simulink model "FULL_HEART_PICTURE"  (R2023a)
settings: Solver=VariableStepAuto  StartTime=0.0  StopTime=60  RelTol=1e-3  AbsTol=1e-3
libraries: fl_lib x33, sh_lib x18, nesl_utility x6, Cardiovascular_lib x4
settings Model: Creator=luca  LastModifiedBy=Syed Abdul Rahman
settings SolverCC: AutoScaleAbsTol=off  ZeroCrossAlgorithm=Adaptive  AlgebraicLoopSolver=TrustRegion
settings DataIOCC: InspectSignalLogs=on
settings DebuggingCC: IgnoredZcDiagnostic=none  UnconnectedInputMsg=warning  UnconnectedOutputMsg=warning  UnconnectedLineMsg=warning  SymbolicDimsDataTypeCodeGenerationDiagnostic=none
settings ModelReferenceCC: EnableRefExpFcnMdlSchedulingChecks=on
settings SFSimCC: CustomCodeUndefinedFunction=UseInterfaceOnly
settings SimscapeCC: SimscapeLogType=all  SimscapeLogSimulationStatistics=on  SimscapeLogDataHistory=10000

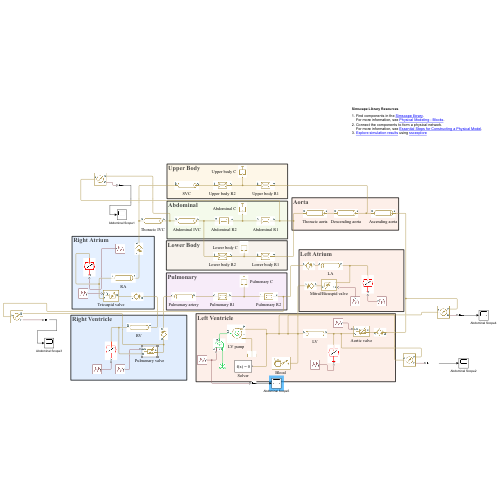
[thumbnail: Simulink's stored preview of the top-level diagram]
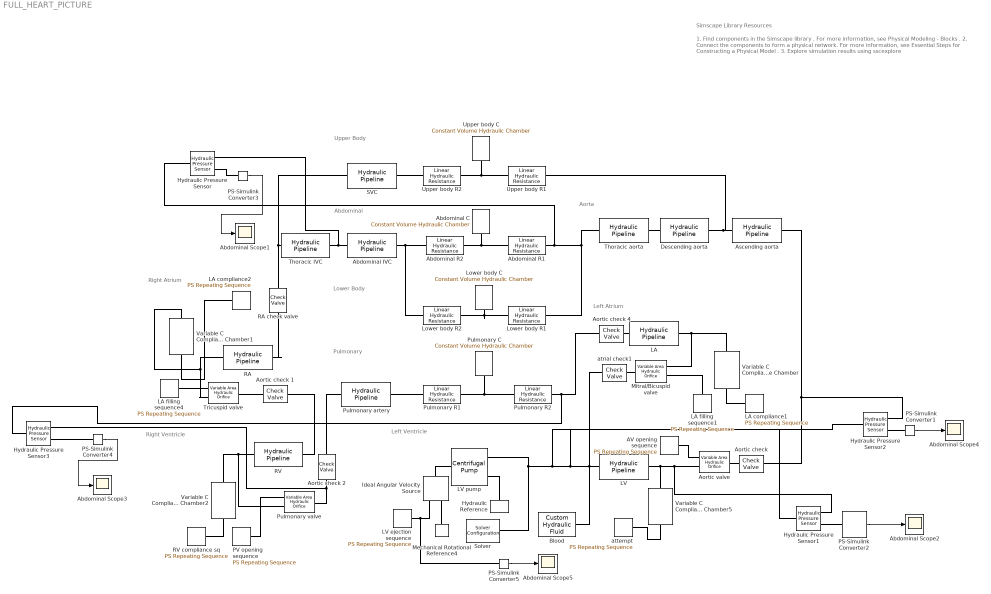
== system FULL_HEART_PICTURE ==
  note: Lower Body
  note: Left Atrium
  note: Right Ventricle
  note: Abdominal
  note: Aorta
  note: 1. Find components in the Simscape library .
      | For more information, see Physical Modeling - Blocks .
      | 2. Connect the components to form a physical network.
      | For more information, see Essential Steps for Constructing a Physical Model .
      | 3. Explore simulation results using sscexplore
  note: Simscape Library Resources
  note: Left Ventricle
  note: Right Atrium
  note: Pulmonary
  note: Upper Body
  AV opening sequence : fl_lib/Physical Signals/Sources/PS Repeating Sequence  y_init=0  offset=0 s  sig_type=2  durations=[0.01 0.01 0.01 0.01 0.01 0.01 0.01 0.01 0.01 0.01 0.01 0.01 0.01 0.01 0.01 0.01 0.01 0.01 0.01 0.01 0.01 0.01 0.01 0.01 0.01 0.01 0.01 0.01 0.01 0.01 0.01 0.01 0.01 0.01 0.01 0.01 0.01 0.01 0.01 0.01 0.01 0.01 0.01 0.01 0.01 0.01 0.01 0.01 0.01 0.01 0.01 0.01 0.01 0.01 0.01 0.01 0.01 0.01 0.01 0.01 0.01 0.01 0.01 0.01 0.01 0.01 0.01 0.01 0.01 0.01 0.01 0.01 0.01 0.01 0.01 0.01 0.01 0.01 0.01 0.01 0.01 0.01 0.01 0.01 0.01 0.01 0.01 0.01 0.01 0.01 0.01 0.01 0.01 0.01 0.01 0.01 0.01 0.01 0.01 0.01] s  y_start="[0.000300000000000000\t0.000300000000000000\t0.000300000000000000\t0.000300000000000000\t0.000300000000000000\t0.000300000000000000\t0.000300000000000000\t0.000300000000000000\t0.000300000000000000\t0.000300000000000000\t0.000300000000000000\t0.000300000000000000\t0.000300000000000000\t0.000300000000000000\t0.000300000000000000\t0.000300000000000000\t0.000300000000000000\t0.000300000000000000\t0.000300000000000000\t0.000300000000000000\t0.000300000000000000\t0.000300000000000000\t0.000300000000000000\t0.000300000000000000\t0.000300000000000000\t0.000300000000000000\t0.000300000000000000\t0.000300000000000000\t0.000300000000000000\t0.000300000000000000\t0.000300000000000000\t0.000300000000000000\t0.000300000000000000\t0.000300000000000000\t0.000300000000000000\t0.000300000000000000\t0.000300000000000000\t0.000300000000000000\t0.000300000000000000\t0.000300000000000000\t0.000300000000000000\t0.000300000000000000\t0.000300000000000000\t0\t0\t0\t0\t0\t0\t0\t0\t0\t0\t0\t0\t0\t0\t0\t0\t0\t0\t0\t0\t0\t0\t0\t0\t0\t0\t0\t0\t0\t0\t0\t0\t0\t0\t0\t0\t0\t0\t0\t0\t0\t0\t0\t0\t0\t0\t0\t0\t0\t0\t0\t0\t0\t0\t0\t0\t0]/3*4"  y_end=1
      settings: InternalSimscapePortConfiguration="{\"Bottom\":[],\"Left\":[],\"Right\":[{\"id\":\"Y\",\"label\":\"Y\",\"type\":\"output\"}],\"Top\":[]}"
  Abdominal C : fl_lib/Hydraulic/Hydraulic Elements/Constant Volume Hydraulic Chamber  ch_sp=2  wall_type=2  ch_volume=1e-4 m^3  d_in=1 cm  length=2570.700637 cm  pr_r_coef=3.6E-08 m/Pa  time_const=0.01 s  k_sh=1.4  pressure_specify=off  pressure_priority=High  pressure=0 Pa  pressure_nominal_specify=off  pressure_nominal_unit=Pa  pressure_nominal_value=1  diameter_incr_specify=off  diameter_incr_priority=High  diameter_incr=0 m  diameter_incr_nominal_specify=off  diameter_incr_nominal_unit=m  diameter_incr_nominal_value=1  flow_rate_specify=off  flow_rate_priority=None  flow_rate=0.001 m^3/s  flow_rate_nominal_specify=off  flow_rate_nominal_unit=m^3/s  flow_rate_nominal_value=1
      settings: InternalSimscapePortConfiguration="{\"Bottom\":[],\"Left\":[{\"id\":\"A\",\"label\":\"\",\"type\":\"foundation.hydraulic.hydraulic\"}],\"Right\":[],\"Top\":[]}"
  Abdominal IVC : sh_lib/Pipelines/Hydraulic Pipeline  cs_type=1  d_in=1.37 cm  area=1e-4 m^2  D_h=1.12e-2 m  s_factor=64  length=17 cm  length_ad=0 m  roughness=15e-6 m  Re_lam=2000  Re_turb=4000  wall_type=2  pr_r_coef=4.39e-6 m/Pa  time_const=0.01 s  k_sh=1.4  initial_pressure=0 Pa
      settings: InternalSimscapePortConfiguration="{\"Bottom\":[],\"Left\":[{\"id\":\"A\",\"label\":\"A\",\"type\":\"foundation.hydraulic.hydraulic\"}],\"Right\":[{\"id\":\"B\",\"label\":\"B\",\"type\":\"foundation.hydraulic.hydraulic\"}],\"Top\":[]}"
  Abdominal R1 : fl_lib/Hydraulic/Hydraulic Elements/Linear Hydraulic Resistance  resistance=2.3e8 Pa/(m^3/s)  q_specify=off  q_priority=None  q=0.001 m^3/s  q_nominal_specify=off  q_nominal_unit=m^3/s  q_nominal_value=1  p_specify=off  p_priority=None  p=0 Pa  p_nominal_specify=off  p_nominal_unit=Pa  p_nominal_value=1
      settings: InternalSimscapePortConfiguration="{\"Bottom\":[],\"Left\":[{\"id\":\"A\",\"label\":\"A\",\"type\":\"foundation.hydraulic.hydraulic\"}],\"Right\":[{\"id\":\"B\",\"label\":\"B\",\"type\":\"foundation.hydraulic.hydraulic\"}],\"Top\":[]}"
  Abdominal R2 : fl_lib/Hydraulic/Hydraulic Elements/Linear Hydraulic Resistance  resistance=0.15e8 Pa/(m^3/s)  q_specify=off  q_priority=None  q=0.001 m^3/s  q_nominal_specify=off  q_nominal_unit=m^3/s  q_nominal_value=1  p_specify=off  p_priority=None  p=0 Pa  p_nominal_specify=off  p_nominal_unit=Pa  p_nominal_value=1
      settings: InternalSimscapePortConfiguration="{\"Bottom\":[],\"Left\":[{\"id\":\"A\",\"label\":\"A\",\"type\":\"foundation.hydraulic.hydraulic\"}],\"Right\":[{\"id\":\"B\",\"label\":\"B\",\"type\":\"foundation.hydraulic.hydraulic\"}],\"Top\":[]}"
  Abdominal Scope{1..5} (5 alike) : Scope
  "Aortic check " : sh_lib/Valves/Directional Valves/Check Valve  area_max=1e-1 m^2  pres_crack=0.01 Pa  pres_max=0.1 Pa  C_d=1  A_leak=1e-12 m^2  lam_spec=1  B_lam=0.999  Re_cr=12  dynamic=0  tau=0.1 s  area_init=1e-12 m^2
      settings: InternalSimscapePortConfiguration="{\"Bottom\":[],\"Left\":[{\"id\":\"A\",\"label\":\"A\",\"type\":\"foundation.hydraulic.hydraulic\"}],\"Right\":[{\"id\":\"B\",\"label\":\"B\",\"type\":\"foundation.hydraulic.hydraulic\"}],\"Top\":[]}"
  Aortic check 1 : sh_lib/Valves/Directional Valves/Check Valve  area_max=1e-1 m^2  pres_crack=0.01 Pa  pres_max=0.1 Pa  C_d=1  A_leak=1e-12 m^2  lam_spec=1  B_lam=0.999  Re_cr=12  dynamic=0  tau=0.1 s  area_init=1e-12 m^2
      settings: InternalSimscapePortConfiguration="{\"Bottom\":[],\"Left\":[{\"id\":\"A\",\"label\":\"A\",\"type\":\"foundation.hydraulic.hydraulic\"}],\"Right\":[{\"id\":\"B\",\"label\":\"B\",\"type\":\"foundation.hydraulic.hydraulic\"}],\"Top\":[]}"
  Aortic check 2 : sh_lib/Valves/Directional Valves/Check Valve  area_max=1e-1 m^2  pres_crack=0.01 Pa  pres_max=0.1 Pa  C_d=1  A_leak=1e-12 m^2  lam_spec=1  B_lam=0.999  Re_cr=12  dynamic=0  tau=0.1 s  area_init=1e-12 m^2
      settings: InternalSimscapePortConfiguration="{\"Bottom\":[],\"Left\":[{\"id\":\"A\",\"label\":\"A\",\"type\":\"foundation.hydraulic.hydraulic\"}],\"Right\":[{\"id\":\"B\",\"label\":\"B\",\"type\":\"foundation.hydraulic.hydraulic\"}],\"Top\":[]}"
  Aortic check 4 : sh_lib/Valves/Directional Valves/Check Valve  area_max=1e-3 m^2  pres_crack=0.01 Pa  pres_max=0.1 Pa  C_d=1  A_leak=1e-12 m^2  lam_spec=1  B_lam=0.999  Re_cr=12  dynamic=0  tau=0.1 s  area_init=1e-12 m^2
      settings: InternalSimscapePortConfiguration="{\"Bottom\":[],\"Left\":[{\"id\":\"A\",\"label\":\"A\",\"type\":\"foundation.hydraulic.hydraulic\"}],\"Right\":[{\"id\":\"B\",\"label\":\"B\",\"type\":\"foundation.hydraulic.hydraulic\"}],\"Top\":[]}"
  Aortic valve : fl_lib/Hydraulic/Hydraulic Elements/Variable Area Hydraulic Orifice  C_d=1  min_area=1e-15 m^2  lam_spec=1  B_lam=0.999  Re_cr=12  q_specify=off  q_priority=None  q=0.001 m^3/s  q_nominal_specify=off  q_nominal_unit=m^3/s  q_nominal_value=1  p_specify=off  p_priority=None  p=0 Pa  p_nominal_specify=off  p_nominal_unit=Pa  p_nominal_value=1
      settings: InternalSimscapePortConfiguration="{\"Bottom\":[],\"Left\":[{\"id\":\"AR\",\"label\":\"AR\",\"type\":\"input\"},{\"id\":\"A\",\"label\":\"A\",\"type\":\"foundation.hydraulic.hydraulic\"}],\"Right\":[{\"id\":\"B\",\"label\":\"B\",\"type\":\"foundation.hydraulic.hydraulic\"}],\"Top\":[]}"
  Ascending aorta : sh_lib/Pipelines/Hydraulic Pipeline  cs_type=1  d_in=2.65 cm  area=1e-4 m^2  D_h=1.12e-2 m  s_factor=64  length=8.8 cm  length_ad=0 m  roughness=15e-6 m  Re_lam=2000  Re_turb=4000  wall_type=2  pr_r_coef=4.5e-7 m/Pa  time_const=0.01 s  k_sh=1.4  initial_pressure=0 Pa
      settings: InternalSimscapePortConfiguration="{\"Bottom\":[],\"Left\":[{\"id\":\"A\",\"label\":\"A\",\"type\":\"foundation.hydraulic.hydraulic\"}],\"Right\":[{\"id\":\"B\",\"label\":\"B\",\"type\":\"foundation.hydraulic.hydraulic\"}],\"Top\":[]}"
  "Blood " : fl_lib/Hydraulic/Hydraulic Utilities/Custom Hydraulic Fluid  density=1060 kg/m^3  viscosity_kin=3.55e-6 m^2/s  bulk=2.2e9 Pa  alpha=0.005  range_error=2
      settings: InternalSimscapePortConfiguration="{\"Bottom\":[],\"Left\":[],\"Right\":[{\"id\":\"G\",\"label\":\"\",\"type\":\"foundation.hydraulic.hydraulic\"}],\"Top\":[]}"
  Descending aorta : sh_lib/Pipelines/Hydraulic Pipeline  cs_type=1  d_in=2.15 cm  area=1e-4 m^2  D_h=1.12e-2 m  s_factor=64  length=6.94 cm  length_ad=0 m  roughness=15e-6 m  Re_lam=2000  Re_turb=4000  wall_type=2  pr_r_coef=1.4e-6 m/Pa  time_const=0.01 s  k_sh=1.4  initial_pressure=0 Pa
      settings: InternalSimscapePortConfiguration="{\"Bottom\":[],\"Left\":[{\"id\":\"A\",\"label\":\"A\",\"type\":\"foundation.hydraulic.hydraulic\"}],\"Right\":[{\"id\":\"B\",\"label\":\"B\",\"type\":\"foundation.hydraulic.hydraulic\"}],\"Top\":[]}"
  Hydraulic Pressure Sensor{,1..3} (4 alike) : fl_lib/Hydraulic/Hydraulic Sensors/Hydraulic Pressure Sensor
  Hydraulic Reference : fl_lib/Hydraulic/Hydraulic Elements/Hydraulic Reference
  Ideal Angular Velocity Source : fl_lib/Mechanical/Mechanical Sources/Ideal Angular Velocity Source
  LA : sh_lib/Pipelines/Hydraulic Pipeline  cs_type=1  d_in=4.8 cm  area=1e-4 m^2  D_h=1.12e-2 m  s_factor=64  length=5 cm  length_ad=0 m  roughness=15e-6 m  Re_lam=2000  Re_turb=4000  wall_type=1  pr_r_coef=5.9e-6 m/Pa  time_const=0.01 s  k_sh=1.4  initial_pressure=0 Pa
      settings: InternalSimscapePortConfiguration="{\"Bottom\":[],\"Left\":[{\"id\":\"A\",\"label\":\"A\",\"type\":\"foundation.hydraulic.hydraulic\"}],\"Right\":[{\"id\":\"B\",\"label\":\"B\",\"type\":\"foundation.hydraulic.hydraulic\"}],\"Top\":[]}"
  LA compliance1 : fl_lib/Physical Signals/Sources/PS Repeating Sequence  y_init=0  offset=0 s  sig_type=2  durations=[0.01 0.01 0.01 0.01 0.01 0.01 0.01 0.01 0.01 0.01 0.01 0.01 0.01 0.01 0.01 0.01 0.01 0.01 0.01 0.01 0.01 0.01 0.01 0.01 0.01 0.01 0.01 0.01 0.01 0.01 0.01 0.01 0.01 0.01 0.01 0.01 0.01 0.01 0.01 0.01 0.01 0.01 0.01 0.01 0.01 0.01 0.01 0.01 0.01 0.01 0.01 0.01 0.01 0.01 0.01 0.01 0.01 0.01 0.01 0.01 0.01 0.01 0.01 0.01 0.01 0.01 0.01 0.01 0.01 0.01 0.01 0.01 0.01 0.01 0.01 0.01 0.01 0.01 0.01 0.01 0.01 0.01 0.01 0.01 0.01 0.01 0.01 0.01 0.01 0.01 0.01 0.01 0.01 0.01 0.01 0.01 0.01 0.01 0.01 0.01] s  y_start="[1.36500000000000e-05\t1.36862500000000e-05\t1.37225000000000e-05\t1.37587500000000e-05\t1.37950000000000e-05\t1.38312500000000e-05\t1.38675000000000e-05\t1.39037500000000e-05\t1.39400000000000e-05\t1.39762500000000e-05\t1.40125000000000e-05\t1.40487500000000e-05\t1.40850000000000e-05\t1.41212500000000e-05\t1.41575000000000e-05\t1.41937500000000e-05\t1.42300000000000e-05\t1.42662500000000e-05\t1.43025000000000e-05\t1.43387500000000e-05\t1.43750000000000e-05\t1.44112500000000e-05\t1.44475000000000e-05\t1.44837500000000e-05\t1.45200000000000e-05\t1.45562500000000e-05\t1.45925000000000e-05\t1.46287500000000e-05\t1.46650000000000e-05\t1.47012500000000e-05\t1.47375000000000e-05\t1.47737500000000e-05\t1.48100000000000e-05\t1.48462500000000e-05\t1.48825000000000e-05\t1.49187500000000e-05\t1.49550000000000e-05\t1.49912500000000e-05\t1.50275000000000e-05\t1.50637500000000e-05\t1.51000000000000e-05\t1.51362500000000e-05\t1.51725000000000e-05\t1.52087500000000e-05\t1.52450000000000e-05\t1.52812500000000e-05\t1.53175000000000e-05\t1.53537500000000e-05\t1.53900000000000e-05\t1.54262500000000e-05\t1.54625000000000e-05\t1.54987500000000e-05\t1.55350000000000e-05\t1.55712500000000e-05\t1.56075000000000e-05\t1.56437500000000e-05\t1.56800000000000e-05\t1.57162500000000e-05\t1.57525000000000e-05\t1.57887500000000e-05\t1.58250000000000e-05\t1.58612500000000e-05\t1.58975000000000e-05\t1.59337500000000e-05\t1.59700000000000e-05\t1.60062500000000e-05\t1.60425000000000e-05\t1.60787500000000e-05\t1.61150000000000e-05\t1.61512500000000e-05\t1.61875000000000e-05\t1.62237500000000e-05\t1.62600000000000e-05\t1.62962500000000e-05\t1.63325000000000e-05\t1.63687500000000e-05\t1.64050000000000e-05\t1.64412500000000e-05\t1.64775000000000e-05\t1.65137500000000e-05\t1.36500000000000e-05\t1.29125270139567e-05\t1.21876723951708e-05\t1.14878386071372e-05\t1.08250000000000e-05\t1.02104979261007e-05\t9.65484668629601e-06\t9.16755362735452e-06\t8.75695646861792e-06\t8.43008064131123e-06\t8.19251908146676e-06\t8.04833653323797e-06\t8.00000000000000e-06\t8.14165729617270e-06\t8.55952589635133e-06\t9.23265212405563e-06\t1.01272826194982e-05\t1.11985568739858e-05\t1.23927567231468e-05\t1.36500000000000e-05]"  y_end=1
      settings: InternalSimscapePortConfiguration="{\"Bottom\":[],\"Left\":[],\"Right\":[{\"id\":\"Y\",\"label\":\"Y\",\"type\":\"output\"}],\"Top\":[]}"
  LA compliance2 : fl_lib/Physical Signals/Sources/PS Repeating Sequence  y_init=0  offset=0 s  sig_type=2  durations=[0.01 0.01 0.01 0.01 0.01 0.01 0.01 0.01 0.01 0.01 0.01 0.01 0.01 0.01 0.01 0.01 0.01 0.01 0.01 0.01 0.01 0.01 0.01 0.01 0.01 0.01 0.01 0.01 0.01 0.01 0.01 0.01 0.01 0.01 0.01 0.01 0.01 0.01 0.01 0.01 0.01 0.01 0.01 0.01 0.01 0.01 0.01 0.01 0.01 0.01 0.01 0.01 0.01 0.01 0.01 0.01 0.01 0.01 0.01 0.01 0.01 0.01 0.01 0.01 0.01 0.01 0.01 0.01 0.01 0.01 0.01 0.01 0.01 0.01 0.01 0.01 0.01 0.01 0.01 0.01 0.01 0.01 0.01 0.01 0.01 0.01 0.01 0.01 0.01 0.01 0.01 0.01 0.01 0.01 0.01 0.01 0.01 0.01 0.01 0.01] s  y_start="[2.18400000000000e-05\t2.18580000000000e-05\t2.18760000000000e-05\t2.18940000000000e-05\t2.19120000000000e-05\t2.19300000000000e-05\t2.19480000000000e-05\t2.19660000000000e-05\t2.19840000000000e-05\t2.20020000000000e-05\t2.20200000000000e-05\t2.20380000000000e-05\t2.20560000000000e-05\t2.20740000000000e-05\t2.20920000000000e-05\t2.21100000000000e-05\t2.21280000000000e-05\t2.21460000000000e-05\t2.21640000000000e-05\t2.21820000000000e-05\t2.22000000000000e-05\t2.22180000000000e-05\t2.22360000000000e-05\t2.22540000000000e-05\t2.22720000000000e-05\t2.22900000000000e-05\t2.23080000000000e-05\t2.23260000000000e-05\t2.23440000000000e-05\t2.23620000000000e-05\t2.23800000000000e-05\t2.23980000000000e-05\t2.24160000000000e-05\t2.24340000000000e-05\t2.24520000000000e-05\t2.24700000000000e-05\t2.24880000000000e-05\t2.25060000000000e-05\t2.25240000000000e-05\t2.25420000000000e-05\t2.25600000000000e-05\t2.25780000000000e-05\t2.25960000000000e-05\t2.26140000000000e-05\t2.26320000000000e-05\t2.26500000000000e-05\t2.26680000000000e-05\t2.26860000000000e-05\t2.27040000000000e-05\t2.27220000000000e-05\t2.27400000000000e-05\t2.27580000000000e-05\t2.27760000000000e-05\t2.27940000000000e-05\t2.28120000000000e-05\t2.28300000000000e-05\t2.28480000000000e-05\t2.28660000000000e-05\t2.28840000000000e-05\t2.29020000000000e-05\t2.29200000000000e-05\t2.29380000000000e-05\t2.29560000000000e-05\t2.29740000000000e-05\t2.29920000000000e-05\t2.30100000000000e-05\t2.30280000000000e-05\t2.30460000000000e-05\t2.30640000000000e-05\t2.30820000000000e-05\t2.31000000000000e-05\t2.31180000000000e-05\t2.31360000000000e-05\t2.31540000000000e-05\t2.31720000000000e-05\t2.31900000000000e-05\t2.32080000000000e-05\t2.32260000000000e-05\t2.32440000000000e-05\t2.32620000000000e-05\t2.18400000000000e-05\t2.14693056140951e-05\t2.11049539119088e-05\t2.07531790520831e-05\t2.04200000000000e-05\t2.01111175416152e-05\t1.98318167414302e-05\t1.95868765135729e-05\t1.93804878532522e-05\t1.92161821276679e-05\t1.90967706533390e-05\t1.90242965936984e-05\t1.90000000000000e-05\t1.90712047294036e-05\t1.92812484151571e-05\t1.96195985897908e-05\t2.00692889627212e-05\t2.06077701809061e-05\t2.12080405475641e-05\t2.18400000000000e-05]"  y_end=1
      settings: InternalSimscapePortConfiguration="{\"Bottom\":[],\"Left\":[],\"Right\":[{\"id\":\"Y\",\"label\":\"Y\",\"type\":\"output\"}],\"Top\":[]}"
  LA filling sequence1 : fl_lib/Physical Signals/Sources/PS Repeating Sequence  y_init=0  offset=0 s  sig_type=2  durations=[0.01 0.01 0.01 0.01 0.01 0.01 0.01 0.01 0.01 0.01 0.01 0.01 0.01 0.01 0.01 0.01 0.01 0.01 0.01 0.01 0.01 0.01 0.01 0.01 0.01 0.01 0.01 0.01 0.01 0.01 0.01 0.01 0.01 0.01 0.01 0.01 0.01 0.01 0.01 0.01 0.01 0.01 0.01 0.01 0.01 0.01 0.01 0.01 0.01 0.01 0.01 0.01 0.01 0.01 0.01 0.01 0.01 0.01 0.01 0.01 0.01 0.01 0.01 0.01 0.01 0.01 0.01 0.01 0.01 0.01 0.01 0.01 0.01 0.01 0.01 0.01 0.01 0.01 0.01 0.01 0.01 0.01 0.01 0.01 0.01 0.01 0.01 0.01 0.01 0.01 0.01 0.01 0.01 0.01 0.01 0.01 0.01 0.01 0.01 0.01] s  y_start="[0\t0\t0\t0\t0\t0\t0\t0\t0\t0\t0\t0\t0\t0\t0\t0\t0\t0\t0\t0\t0\t0\t0\t0\t0\t0\t0\t0\t0\t0\t0\t0\t0\t0\t0\t0\t0\t0\t0\t0\t0\t0\t0\t0\t0\t0.000420000000000000\t0.000420000000000000\t0.000420000000000000\t0.000420000000000000\t0.000420000000000000\t0.000420000000000000\t0.000420000000000000\t0.000420000000000000\t0.000420000000000000\t0.000420000000000000\t0.000420000000000000\t0.000420000000000000\t0.000420000000000000\t0.000420000000000000\t0.000420000000000000\t0.000420000000000000\t0.000420000000000000\t0.000420000000000000\t0.000420000000000000\t0.000420000000000000\t0.000420000000000000\t0.000420000000000000\t0.000420000000000000\t0.000420000000000000\t0.000420000000000000\t0.000420000000000000\t0.000420000000000000\t0.000420000000000000\t0.000420000000000000\t0.000420000000000000\t0.000420000000000000\t0.000420000000000000\t0.000420000000000000\t0.000420000000000000\t0.000420000000000000\t0.000420000000000000\t0.000420000000000000\t0.000420000000000000\t0.000420000000000000\t0.000420000000000000\t0.000420000000000000\t0.000420000000000000\t0.000420000000000000\t0.000420000000000000\t0.000420000000000000\t0.000420000000000000\t0.000420000000000000\t0.000420000000000000\t0.000420000000000000\t0.000420000000000000\t0.000420000000000000\t0.000420000000000000\t0.000420000000000000\t0.000420000000000000\t0.000420000000000000]"  y_end=1
      settings: InternalSimscapePortConfiguration="{\"Bottom\":[],\"Left\":[],\"Right\":[{\"id\":\"Y\",\"label\":\"Y\",\"type\":\"output\"}],\"Top\":[]}"
  LA filling sequence4 : fl_lib/Physical Signals/Sources/PS Repeating Sequence  y_init=0  offset=0 s  sig_type=2  durations=[0.01 0.01 0.01 0.01 0.01 0.01 0.01 0.01 0.01 0.01 0.01 0.01 0.01 0.01 0.01 0.01 0.01 0.01 0.01 0.01 0.01 0.01 0.01 0.01 0.01 0.01 0.01 0.01 0.01 0.01 0.01 0.01 0.01 0.01 0.01 0.01 0.01 0.01 0.01 0.01 0.01 0.01 0.01 0.01 0.01 0.01 0.01 0.01 0.01 0.01 0.01 0.01 0.01 0.01 0.01 0.01 0.01 0.01 0.01 0.01 0.01 0.01 0.01 0.01 0.01 0.01 0.01 0.01 0.01 0.01 0.01 0.01 0.01 0.01 0.01 0.01 0.01 0.01 0.01 0.01 0.01 0.01 0.01 0.01 0.01 0.01 0.01 0.01 0.01 0.01 0.01 0.01 0.01 0.01 0.01 0.01 0.01 0.01 0.01 0.01] s  y_start="[0\t0\t0\t0\t0\t0\t0\t0\t0\t0\t0\t0\t0\t0\t0\t0\t0\t0\t0\t0\t0\t0\t0\t0\t0\t0\t0\t0\t0\t0\t0\t0\t0\t0\t0\t0\t0\t0\t0\t0\t0\t0\t0\t0\t0\t0.000500000000000000\t0.000500000000000000\t0.000500000000000000\t0.000500000000000000\t0.000500000000000000\t0.000500000000000000\t0.000500000000000000\t0.000500000000000000\t0.000500000000000000\t0.000500000000000000\t0.000500000000000000\t0.000500000000000000\t0.000500000000000000\t0.000500000000000000\t0.000500000000000000\t0.000500000000000000\t0.000500000000000000\t0.000500000000000000\t0.000500000000000000\t0.000500000000000000\t0.000500000000000000\t0.000500000000000000\t0.000500000000000000\t0.000500000000000000\t0.000500000000000000\t0.000500000000000000\t0.000500000000000000\t0.000500000000000000\t0.000500000000000000\t0.000500000000000000\t0.000500000000000000\t0.000500000000000000\t0.000500000000000000\t0.000500000000000000\t0.000500000000000000\t0.000500000000000000\t0.000500000000000000\t0.000500000000000000\t0.000500000000000000\t0.000500000000000000\t0.000500000000000000\t0.000500000000000000\t0.000500000000000000\t0.000500000000000000\t0.000500000000000000\t0.000500000000000000\t0.000500000000000000\t0.000500000000000000\t0.000500000000000000\t0.000500000000000000\t0.000500000000000000\t0.000500000000000000\t0.000500000000000000\t0.000500000000000000\t0.000500000000000000]"  y_end=1
      settings: InternalSimscapePortConfiguration="{\"Bottom\":[],\"Left\":[],\"Right\":[{\"id\":\"Y\",\"label\":\"Y\",\"type\":\"output\"}],\"Top\":[]}"
  LV : sh_lib/Pipelines/Hydraulic Pipeline  cs_type=1  d_in=4.4 cm  area=1e-4 m^2  D_h=1.12e-2 m  s_factor=64  length=7 cm  length_ad=0 m  roughness=15e-6 m  Re_lam=2000  Re_turb=4000  wall_type=1  pr_r_coef=3.8e-7 m/Pa  time_const=0.01 s  k_sh=1.4  initial_pressure=0 Pa
      settings: InternalSimscapePortConfiguration="{\"Bottom\":[],\"Left\":[{\"id\":\"A\",\"label\":\"A\",\"type\":\"foundation.hydraulic.hydraulic\"}],\"Right\":[{\"id\":\"B\",\"label\":\"B\",\"type\":\"foundation.hydraulic.hydraulic\"}],\"Top\":[]}"
  LV ejection sequence : fl_lib/Physical Signals/Sources/PS Repeating Sequence  y_init=0  offset=0 s  sig_type=2  durations=[0.01 0.01 0.01 0.01 0.01 0.01 0.01 0.01 0.01 0.01 0.01 0.01 0.01 0.01 0.01 0.01 0.01 0.01 0.01 0.01 0.01 0.01 0.01 0.01 0.01 0.01 0.01 0.01 0.01 0.01 0.01 0.01 0.01 0.01 0.01 0.01 0.01 0.01 0.01 0.01 0.01 0.01 0.01 0.01 0.01 0.01 0.01 0.01 0.01 0.01 0.01 0.01 0.01 0.01 0.01 0.01 0.01 0.01 0.01 0.01 0.01 0.01 0.01 0.01 0.01 0.01 0.01 0.01 0.01 0.01 0.01 0.01 0.01 0.01 0.01 0.01 0.01 0.01 0.01 0.01 0.01 0.01 0.01 0.01 0.01 0.01 0.01 0.01 0.01 0.01 0.01 0.01 0.01 0.01 0.01 0.01 0.01 0.01 0.01 0.01] s  y_start=[26.89 53.68 80.24 106.49 132.30 157.58 182.23 206.15 229.23 251.39 272.54 292.59 311.47 329.09 345.38 360.28 373.74 385.68 396.08 404.88 412.05 417.56 421.39 423.52 423.95 422.670 419.68 415.01 408.67 400.68 391.08 379.90 367.19 353.01 337.4 320.44 302.18 282.71 262.1 240.43 217.80 194.29 169.99 145.02 119.45 93.41 66.99 40.3 13.45 0 0 0 0 0 0 0 0 0 0 0 0 0 0 0 0 0 0 0 0 0 0 0 0 0 0 0 0 0 0 0 0 0 0 0 0 0 0 0 0 0 0 0 0 0 0 0 0 0 0 0]*1.15e-1  y_end=1
      settings: InternalSimscapePortConfiguration="{\"Bottom\":[],\"Left\":[],\"Right\":[{\"id\":\"Y\",\"label\":\"Y\",\"type\":\"output\"}],\"Top\":[]}"
  LV pump : sh_lib/Pumps and Motors/Centrifugal Pump  mdl_type=1  c_1=326.8 Pa/(kg/m^3)  c_2=3.104e4 Pa*s/kg  c_3=1.097e7 Pa*s^2/(kg*m^3)  c_4=2.136e5 Pa*s^2/(kg*m^3)  c_f=0.8  design_del=130 lpm  ref_velocity=1770 rpm  ref_density=1060 kg/m^3  leak_resistance=7e6 Pa/(m^3/s)  T_const=0.1 N*m  trq_press_coeff=0.1e-5 N*m/Pa  pump_del_1D=[0, 28, 90, 130, 154, 182] lpm  press_diff_1D=[2.6, 2.4, 2, 1.6, 1.2, .8] bar  pump_del_power_1D=[0, 20, 40, 60, 80, 100, 120, 140, 160] lpm  power_1D=[220, 280, 310, 360, 390, 420, 480, 500, 550] W  pump_vel_2D=[3200, 3300, 3400, 3500] rpm  pump_del_2D=[0, 50, 100, 150, 200, 250, 300, 350] lpm  press_diff_2D=[8.3, 8.8, 9.3, 9.9; 7.8, 8.3, 8.8, 9.4; 7.2, 7.6, 8.2, 8.7; 6.5, 7, 7.5, 8; 5.6, 6.1, 6.6, 7.1; 4.7, 5.2, 5.7, 6.2; 3.4, 4, 4.4, 4.9; 2.3, 2.7, 3.4, 3.6] bar  pump_del_power_2D=[0, 50, 100, 150, 200, 250, 300, 350] lpm  power_2D=[1223, 1341, 1467, 1600; 1414, 1551, 1696, 1850; 1636, 1794, 1962, 2140; 1941, 2129, 2326, 2540; 2224, 2439, 2660, 2910; 2453, 2691, 2947, 3210; 2757, 3024, 3307, 3608; 2945, 3230, 3533, 3854] W  omega_threshold=1e-9 rad/s  interp_method=1  extrap_method=1
      settings: InternalSimscapePortConfiguration="{\"Bottom\":[],\"Left\":[{\"id\":\"S\",\"label\":\"S\",\"type\":\"foundation.mechanical.rotational.rotational\"}],\"Right\":[{\"id\":\"P\",\"label\":\"P\",\"type\":\"foundation.hydraulic.hydraulic\"},{\"id\":\"T\",\"label\":\"T\",\"type\":\"foundation.hydraulic.hydraulic\"}],\"Top\":[]}"
  Lower body C : fl_lib/Hydraulic/Hydraulic Elements/Constant Volume Hydraulic Chamber  ch_sp=2  wall_type=2  ch_volume=1e-4 m^3  d_in=1 cm  length=648.4076433 cm  pr_r_coef=4.1E-08 m/Pa  time_const=0.01 s  k_sh=1.4  pressure_specify=off  pressure_priority=High  pressure=0 Pa  pressure_nominal_specify=off  pressure_nominal_unit=Pa  pressure_nominal_value=1  diameter_incr_specify=off  diameter_incr_priority=High  diameter_incr=0 m  diameter_incr_nominal_specify=off  diameter_incr_nominal_unit=m  diameter_incr_nominal_value=1  flow_rate_specify=off  flow_rate_priority=None  flow_rate=0.001 m^3/s  flow_rate_nominal_specify=off  flow_rate_nominal_unit=m^3/s  flow_rate_nominal_value=1
      settings: InternalSimscapePortConfiguration="{\"Bottom\":[],\"Left\":[{\"id\":\"A\",\"label\":\"\",\"type\":\"foundation.hydraulic.hydraulic\"}],\"Right\":[],\"Top\":[]}"
  Lower body R1 : fl_lib/Hydraulic/Hydraulic Elements/Linear Hydraulic Resistance  resistance=4.79e8 Pa/(m^3/s)  q_specify=off  q_priority=None  q=0.001 m^3/s  q_nominal_specify=off  q_nominal_unit=m^3/s  q_nominal_value=1  p_specify=off  p_priority=None  p=0 Pa  p_nominal_specify=off  p_nominal_unit=Pa  p_nominal_value=1
      settings: InternalSimscapePortConfiguration="{\"Bottom\":[],\"Left\":[{\"id\":\"A\",\"label\":\"A\",\"type\":\"foundation.hydraulic.hydraulic\"}],\"Right\":[{\"id\":\"B\",\"label\":\"B\",\"type\":\"foundation.hydraulic.hydraulic\"}],\"Top\":[]}"
  Lower body R2 : fl_lib/Hydraulic/Hydraulic Elements/Linear Hydraulic Resistance  resistance=0.4e8 Pa/(m^3/s)  q_specify=off  q_priority=None  q=0.001 m^3/s  q_nominal_specify=off  q_nominal_unit=m^3/s  q_nominal_value=1  p_specify=off  p_priority=None  p=0 Pa  p_nominal_specify=off  p_nominal_unit=Pa  p_nominal_value=1
      settings: InternalSimscapePortConfiguration="{\"Bottom\":[],\"Left\":[{\"id\":\"A\",\"label\":\"A\",\"type\":\"foundation.hydraulic.hydraulic\"}],\"Right\":[{\"id\":\"B\",\"label\":\"B\",\"type\":\"foundation.hydraulic.hydraulic\"}],\"Top\":[]}"
  Mechanical Rotational Reference4 : fl_lib/Mechanical/Rotational Elements/Mechanical Rotational Reference
  Mitral/Bicuspid valve : fl_lib/Hydraulic/Hydraulic Elements/Variable Area Hydraulic Orifice  C_d=1  min_area=1e-15 m^2  lam_spec=1  B_lam=0.999  Re_cr=12  q_specify=off  q_priority=None  q=0.001 m^3/s  q_nominal_specify=off  q_nominal_unit=m^3/s  q_nominal_value=1  p_specify=off  p_priority=None  p=0 Pa  p_nominal_specify=off  p_nominal_unit=Pa  p_nominal_value=1
      settings: InternalSimscapePortConfiguration="{\"Bottom\":[],\"Left\":[{\"id\":\"AR\",\"label\":\"AR\",\"type\":\"input\"},{\"id\":\"A\",\"label\":\"A\",\"type\":\"foundation.hydraulic.hydraulic\"}],\"Right\":[{\"id\":\"B\",\"label\":\"B\",\"type\":\"foundation.hydraulic.hydraulic\"}],\"Top\":[]}"
  PS-Simulink Converter{1..5} (5 alike) : nesl_utility/PS-Simulink Converter  PhysicalDomain=network_engine_domain  SubClassName=ps_output  LeftPortType=input  RightPortType=output  PseudoPeriodic=off  Frequencies=[]  VectorFormat=1-D array  Unit=inherit  AffineConversion=off
  PV opening sequence : fl_lib/Physical Signals/Sources/PS Repeating Sequence  y_init=0  offset=0 s  sig_type=2  durations=[0.01 0.01 0.01 0.01 0.01 0.01 0.01 0.01 0.01 0.01 0.01 0.01 0.01 0.01 0.01 0.01 0.01 0.01 0.01 0.01 0.01 0.01 0.01 0.01 0.01 0.01 0.01 0.01 0.01 0.01 0.01 0.01 0.01 0.01 0.01 0.01 0.01 0.01 0.01 0.01 0.01 0.01 0.01 0.01 0.01 0.01 0.01 0.01 0.01 0.01 0.01 0.01 0.01 0.01 0.01 0.01 0.01 0.01 0.01 0.01 0.01 0.01 0.01 0.01 0.01 0.01 0.01 0.01 0.01 0.01 0.01 0.01 0.01 0.01 0.01 0.01 0.01 0.01 0.01 0.01 0.01 0.01 0.01 0.01 0.01 0.01 0.01 0.01 0.01 0.01 0.01 0.01 0.01 0.01 0.01 0.01 0.01 0.01 0.01 0.01] s  y_start="[0.000300000000000000\t0.000300000000000000\t0.000300000000000000\t0.000300000000000000\t0.000300000000000000\t0.000300000000000000\t0.000300000000000000\t0.000300000000000000\t0.000300000000000000\t0.000300000000000000\t0.000300000000000000\t0.000300000000000000\t0.000300000000000000\t0.000300000000000000\t0.000300000000000000\t0.000300000000000000\t0.000300000000000000\t0.000300000000000000\t0.000300000000000000\t0.000300000000000000\t0.000300000000000000\t0.000300000000000000\t0.000300000000000000\t0.000300000000000000\t0.000300000000000000\t0.000300000000000000\t0.000300000000000000\t0.000300000000000000\t0.000300000000000000\t0.000300000000000000\t0.000300000000000000\t0.000300000000000000\t0.000300000000000000\t0.000300000000000000\t0.000300000000000000\t0.000300000000000000\t0.000300000000000000\t0.000300000000000000\t0.000300000000000000\t0.000300000000000000\t0.000300000000000000\t0.000300000000000000\t0.000300000000000000\t0.000300000000000000\t0.000300000000000000\t\t0.000300000000000000\t0.000300000000000000\t0.000300000000000000\t0.000300000000000000\t0.000300000000000000\t0.000300000000000000\t0.000300000000000000\t0.000300000000000000\t0\t0\t0\t0\t0\t0\t0\t0\t0\t0\t0\t0\t0\t0\t0\t0\t0\t0\t0\t0\t0\t0\t0\t0\t0\t0\t0\t0\t0\t0\t0\t0\t0\t0\t0\t0\t0\t0\t0\t0\t0\t0\t0 0 0 0 0]/3*5"  y_end=1
      settings: InternalSimscapePortConfiguration="{\"Bottom\":[],\"Left\":[],\"Right\":[{\"id\":\"Y\",\"label\":\"Y\",\"type\":\"output\"}],\"Top\":[]}"
  Pulmonary C : fl_lib/Hydraulic/Hydraulic Elements/Constant Volume Hydraulic Chamber  ch_sp=2  wall_type=2  ch_volume=1e-4 m^3  d_in=1 cm  length=702.4 cm  pr_r_coef=6e-7 m/Pa  time_const=0.01 s  k_sh=1.4  pressure_specify=off  pressure_priority=High  pressure=0 Pa  pressure_nominal_specify=off  pressure_nominal_unit=Pa  pressure_nominal_value=1  diameter_incr_specify=off  diameter_incr_priority=High  diameter_incr=0 m  diameter_incr_nominal_specify=off  diameter_incr_nominal_unit=m  diameter_incr_nominal_value=1  flow_rate_specify=off  flow_rate_priority=None  flow_rate=0.001 m^3/s  flow_rate_nominal_specify=off  flow_rate_nominal_unit=m^3/s  flow_rate_nominal_value=1
      settings: InternalSimscapePortConfiguration="{\"Bottom\":[],\"Left\":[{\"id\":\"A\",\"label\":\"\",\"type\":\"foundation.hydraulic.hydraulic\"}],\"Right\":[],\"Top\":[]}"
  Pulmonary R1 : fl_lib/Hydraulic/Hydraulic Elements/Linear Hydraulic Resistance  resistance=0.5e7 Pa/(m^3/s)  q_specify=off  q_priority=None  q=0.001 m^3/s  q_nominal_specify=off  q_nominal_unit=m^3/s  q_nominal_value=1  p_specify=off  p_priority=None  p=0 Pa  p_nominal_specify=off  p_nominal_unit=Pa  p_nominal_value=1
      settings: InternalSimscapePortConfiguration="{\"Bottom\":[],\"Left\":[{\"id\":\"A\",\"label\":\"A\",\"type\":\"foundation.hydraulic.hydraulic\"}],\"Right\":[{\"id\":\"B\",\"label\":\"B\",\"type\":\"foundation.hydraulic.hydraulic\"}],\"Top\":[]}"
  Pulmonary R2 : fl_lib/Hydraulic/Hydraulic Elements/Linear Hydraulic Resistance  resistance=0.05e7 Pa/(m^3/s)  q_specify=off  q_priority=None  q=0.001 m^3/s  q_nominal_specify=off  q_nominal_unit=m^3/s  q_nominal_value=1  p_specify=off  p_priority=None  p=0 Pa  p_nominal_specify=off  p_nominal_unit=Pa  p_nominal_value=1
      settings: InternalSimscapePortConfiguration="{\"Bottom\":[],\"Left\":[{\"id\":\"A\",\"label\":\"A\",\"type\":\"foundation.hydraulic.hydraulic\"}],\"Right\":[{\"id\":\"B\",\"label\":\"B\",\"type\":\"foundation.hydraulic.hydraulic\"}],\"Top\":[]}"
  Pulmonary artery : sh_lib/Pipelines/Hydraulic Pipeline  cs_type=1  d_in=3 cm  area=1e-4 m^2  D_h=1.12e-2 m  s_factor=64  length=5 cm  length_ad=0 m  roughness=15e-6 m  Re_lam=2000  Re_turb=4000  wall_type=2  pr_r_coef=2.2e-7 m/Pa  time_const=0.01 s  k_sh=1.4  initial_pressure=0 Pa
      settings: InternalSimscapePortConfiguration="{\"Bottom\":[],\"Left\":[{\"id\":\"A\",\"label\":\"A\",\"type\":\"foundation.hydraulic.hydraulic\"}],\"Right\":[{\"id\":\"B\",\"label\":\"B\",\"type\":\"foundation.hydraulic.hydraulic\"}],\"Top\":[]}"
  Pulmonary valve : fl_lib/Hydraulic/Hydraulic Elements/Variable Area Hydraulic Orifice  C_d=1  min_area=1e-15 m^2  lam_spec=1  B_lam=0.999  Re_cr=12  q_specify=off  q_priority=None  q=0.001 m^3/s  q_nominal_specify=off  q_nominal_unit=m^3/s  q_nominal_value=1  p_specify=off  p_priority=None  p=0 Pa  p_nominal_specify=off  p_nominal_unit=Pa  p_nominal_value=1
      settings: InternalSimscapePortConfiguration="{\"Bottom\":[],\"Left\":[{\"id\":\"AR\",\"label\":\"AR\",\"type\":\"input\"},{\"id\":\"A\",\"label\":\"A\",\"type\":\"foundation.hydraulic.hydraulic\"}],\"Right\":[{\"id\":\"B\",\"label\":\"B\",\"type\":\"foundation.hydraulic.hydraulic\"}],\"Top\":[]}"
  RA : sh_lib/Pipelines/Hydraulic Pipeline  cs_type=1  d_in=5.6 cm  area=1e-4 m^2  D_h=1.12e-2 m  s_factor=64  length=5 cm  length_ad=0 m  roughness=15e-6 m  Re_lam=2000  Re_turb=4000  wall_type=1  pr_r_coef=5.9e-6 m/Pa  time_const=0.01 s  k_sh=1.4  initial_pressure=0 Pa
      settings: InternalSimscapePortConfiguration="{\"Bottom\":[],\"Left\":[{\"id\":\"A\",\"label\":\"A\",\"type\":\"foundation.hydraulic.hydraulic\"}],\"Right\":[{\"id\":\"B\",\"label\":\"B\",\"type\":\"foundation.hydraulic.hydraulic\"}],\"Top\":[]}"
  RA check valve : sh_lib/Valves/Directional Valves/Check Valve  area_max=1e-1 m^2  pres_crack=0.01 Pa  pres_max=0.1 Pa  C_d=1  A_leak=1e-12 m^2  lam_spec=1  B_lam=0.999  Re_cr=12  dynamic=0  tau=0.1 s  area_init=1e-12 m^2
      settings: InternalSimscapePortConfiguration="{\"Bottom\":[],\"Left\":[{\"id\":\"A\",\"label\":\"A\",\"type\":\"foundation.hydraulic.hydraulic\"}],\"Right\":[{\"id\":\"B\",\"label\":\"B\",\"type\":\"foundation.hydraulic.hydraulic\"}],\"Top\":[]}"
  RV : sh_lib/Pipelines/Hydraulic Pipeline  cs_type=1  d_in=5 cm  area=1e-4 m^2  D_h=1.12e-2 m  s_factor=64  length=7.5 cm  length_ad=0 m  roughness=15e-6 m  Re_lam=2000  Re_turb=4000  wall_type=1  pr_r_coef=3.8e-7 m/Pa  time_const=0.01 s  k_sh=1.4  initial_pressure=0 Pa
      settings: InternalSimscapePortConfiguration="{\"Bottom\":[],\"Left\":[{\"id\":\"A\",\"label\":\"A\",\"type\":\"foundation.hydraulic.hydraulic\"}],\"Right\":[{\"id\":\"B\",\"label\":\"B\",\"type\":\"foundation.hydraulic.hydraulic\"}],\"Top\":[]}"
  RV compliance sq : fl_lib/Physical Signals/Sources/PS Repeating Sequence  y_init=0  offset=0 s  sig_type=2  durations=[0.01 0.01 0.01 0.01 0.01 0.01 0.01 0.01 0.01 0.01 0.01 0.01 0.01 0.01 0.01 0.01 0.01 0.01 0.01 0.01 0.01 0.01 0.01 0.01 0.01 0.01 0.01 0.01 0.01 0.01 0.01 0.01 0.01 0.01 0.01 0.01 0.01 0.01 0.01 0.01 0.01 0.01 0.01 0.01 0.01 0.01 0.01 0.01 0.01 0.01 0.01 0.01 0.01 0.01 0.01 0.01 0.01 0.01 0.01 0.01 0.01 0.01 0.01 0.01 0.01 0.01 0.01 0.01 0.01 0.01 0.01 0.01 0.01 0.01 0.01 0.01 0.01 0.01 0.01 0.01 0.01 0.01 0.01 0.01 0.01 0.01 0.01 0.01 0.01 0.01 0.01 0.01 0.01 0.01 0.01 0.01 0.01 0.01 0.01 0.01] s  y_start="[5.50000000000000e-05\t5.26294018607136e-05\t5.02685450176733e-05\t4.79271307380492e-05\t4.56147803953482e-05\t4.33409959331260e-05\t4.11151208194632e-05\t3.89463016526504e-05\t3.68434505758543e-05\t3.48152086552097e-05\t3.28699103718250e-05\t3.10155493736118e-05\t2.92597456276710e-05\t2.76097141082133e-05\t2.60722351486829e-05\t2.46536265799126e-05\t2.33597177688022e-05\t2.21958256641990e-05\t2.11667329484149e-05\t2.02766683841589e-05\t1.95292894376436e-05\t1.89276672492725e-05\t1.84742740136653e-05\t1.81709728208797e-05\t1.80190100005745e-05\t1.80190100005745e-05\t1.81709728208797e-05\t1.84742740136653e-05\t1.89276672492725e-05\t1.95292894376436e-05\t2.02766683841589e-05\t2.11667329484149e-05\t2.21958256641990e-05\t2.33597177688022e-05\t2.46536265799126e-05\t2.60722351486829e-05\t2.76097141082133e-05\t2.92597456276710e-05\t3.10155493736118e-05\t3.28699103718250e-05\t3.48152086552097e-05\t3.68434505758543e-05\t3.89463016526503e-05\t4.11151208194631e-05\t4.33409959331260e-05\t4.56147803953482e-05\t4.79271307380492e-05\t5.02685450176733e-05\t5.26294018607136e-05\t5.50000000000000e-05\t5.50000000000000e-05\t5.50000000000000e-05\t5.50000000000000e-05\t5.50000000000000e-05\t5.50000000000000e-05\t5.50000000000000e-05\t5.50000000000000e-05\t5.50000000000000e-05\t5.50000000000000e-05\t5.50000000000000e-05\t5.50000000000000e-05\t5.50000000000000e-05\t5.50000000000000e-05\t5.50000000000000e-05\t5.50000000000000e-05\t5.50000000000000e-05\t5.50000000000000e-05\t5.50000000000000e-05\t5.50000000000000e-05\t5.50000000000000e-05\t5.50000000000000e-05\t5.50000000000000e-05\t5.50000000000000e-05\t5.50000000000000e-05\t5.50000000000000e-05\t5.50000000000000e-05\t5.50000000000000e-05\t5.50000000000000e-05\t5.50000000000000e-05\t5.50000000000000e-05\t5.50000000000000e-05\t5.50000000000000e-05\t5.50000000000000e-05\t5.50000000000000e-05\t5.50000000000000e-05\t5.50000000000000e-05\t5.50000000000000e-05\t5.50000000000000e-05\t5.50000000000000e-05\t5.50000000000000e-05\t5.50000000000000e-05\t5.50000000000000e-05\t5.50000000000000e-05\t5.50000000000000e-05\t5.50000000000000e-05\t5.50000000000000e-05\t5.50000000000000e-05\t5.50000000000000e-05\t5.50000000000000e-05\t5.50000000000000e-05]"  y_end=1
      settings: InternalSimscapePortConfiguration="{\"Bottom\":[],\"Left\":[],\"Right\":[{\"id\":\"Y\",\"label\":\"Y\",\"type\":\"output\"}],\"Top\":[]}"
  SVC : sh_lib/Pipelines/Hydraulic Pipeline  cs_type=1  d_in=2.1 cm  area=1e-4 m^2  D_h=1.12e-2 m  s_factor=64  length=7.1 cm  length_ad=0 m  roughness=15e-6 m  Re_lam=2000  Re_turb=4000  wall_type=2  pr_r_coef=5e-6 m/Pa  time_const=0.01 s  k_sh=1.4  initial_pressure=0 Pa
      settings: InternalSimscapePortConfiguration="{\"Bottom\":[],\"Left\":[{\"id\":\"A\",\"label\":\"A\",\"type\":\"foundation.hydraulic.hydraulic\"}],\"Right\":[{\"id\":\"B\",\"label\":\"B\",\"type\":\"foundation.hydraulic.hydraulic\"}],\"Top\":[]}"
  Solver : nesl_utility/Solver Configuration  PhysicalDomain=network_engine_domain  SubClassName=solver  LeftPortType=input  RightPortType=generic  Tones=[]  Harmonics=[]  SimulateNoise=off  Profile=off  UseLocalSampling=off  EnableSwitchedLinearOptims=on  FrequencyDomain=off  UseCCode=off  RelTol=0.001  AbsTol=1e-06  MinStep=1e-09  ToWorkspace=off  RevertToSquareIcSolve=off  NumHomotopyIterations=100  PhasorMode=off  PhasorModeNumHarmonics=1  ConsistencySolver=NEWTON_FTOL  IndexReductionMethod=DerivativeReplacement  DoDC=off  ResidualTolerance=1e-09  ConsistencyTolSource=GLOBAL  ConsistencyAbsTol=0.001  ConsistencyRelTol=0.001  ConsistencyTolFactor=0.001  UseLocalSolver=off  LocalSolverChoice=NE_BACKWARD_EULER_ADVANCER  ResolveIndetEquations=on  FunctionEvalNumThread=1  LocalSolverSampleTime=0.001  DoFixedCost=off  MaxNonlinIter=3  MaxModeIter=2  ComputeImpulses=off  ImpulseIterations=2  LinearAlgebra=auto  LinearAlgebraNumThread=0  EquationFormulation=NE_TIME_EF  DelaysMemoryBudget=1024  AutomaticFiltering=on  FilteringTimeConstant=0.00001  PartitionStorageMethod=AS_NEEDED  PartitionMemoryBudget=1024  PartitionMethod=ROBUST
  Thoracic IVC : sh_lib/Pipelines/Hydraulic Pipeline  cs_type=1  d_in=1.37 cm  area=1e-4 m^2  D_h=1.12e-2 m  s_factor=64  length=2.5 cm  length_ad=0 m  roughness=15e-6 m  Re_lam=2000  Re_turb=4000  wall_type=2  pr_r_coef=6.37e-7 m/Pa  time_const=0.01 s  k_sh=1.4  initial_pressure=0 Pa
      settings: InternalSimscapePortConfiguration="{\"Bottom\":[],\"Left\":[{\"id\":\"A\",\"label\":\"A\",\"type\":\"foundation.hydraulic.hydraulic\"}],\"Right\":[{\"id\":\"B\",\"label\":\"B\",\"type\":\"foundation.hydraulic.hydraulic\"}],\"Top\":[]}"
  Thoracic aorta : sh_lib/Pipelines/Hydraulic Pipeline  cs_type=1  d_in=1.92 cm  area=1e-4 m^2  D_h=1.12e-2 m  s_factor=64  length=33.2 cm  length_ad=0 m  roughness=15e-6 m  Re_lam=2000  Re_turb=4000  wall_type=2  pr_r_coef=3.3e-7 m/Pa  time_const=0.01 s  k_sh=1.4  initial_pressure=0 Pa
      settings: InternalSimscapePortConfiguration="{\"Bottom\":[],\"Left\":[{\"id\":\"A\",\"label\":\"A\",\"type\":\"foundation.hydraulic.hydraulic\"}],\"Right\":[{\"id\":\"B\",\"label\":\"B\",\"type\":\"foundation.hydraulic.hydraulic\"}],\"Top\":[]}"
  Tricuspid valve : fl_lib/Hydraulic/Hydraulic Elements/Variable Area Hydraulic Orifice  C_d=1  min_area=1e-15 m^2  lam_spec=1  B_lam=0.999  Re_cr=12  q_specify=off  q_priority=None  q=0.001 m^3/s  q_nominal_specify=off  q_nominal_unit=m^3/s  q_nominal_value=1  p_specify=off  p_priority=None  p=0 Pa  p_nominal_specify=off  p_nominal_unit=Pa  p_nominal_value=1
      settings: InternalSimscapePortConfiguration="{\"Bottom\":[],\"Left\":[{\"id\":\"AR\",\"label\":\"AR\",\"type\":\"input\"},{\"id\":\"A\",\"label\":\"A\",\"type\":\"foundation.hydraulic.hydraulic\"}],\"Right\":[{\"id\":\"B\",\"label\":\"B\",\"type\":\"foundation.hydraulic.hydraulic\"}],\"Top\":[]}"
  Upper body C : fl_lib/Hydraulic/Hydraulic Elements/Constant Volume Hydraulic Chamber  ch_sp=2  wall_type=2  ch_volume=1e-4 m^3  d_in=1 cm  length=1131.210191 cm  pr_r_coef=6.7E-08 m/Pa  time_const=0.01 s  k_sh=1.4  pressure_specify=off  pressure_priority=High  pressure=0 Pa  pressure_nominal_specify=off  pressure_nominal_unit=Pa  pressure_nominal_value=1  diameter_incr_specify=off  diameter_incr_priority=High  diameter_incr=0 m  diameter_incr_nominal_specify=off  diameter_incr_nominal_unit=m  diameter_incr_nominal_value=1  flow_rate_specify=off  flow_rate_priority=None  flow_rate=0.001 m^3/s  flow_rate_nominal_specify=off  flow_rate_nominal_unit=m^3/s  flow_rate_nominal_value=1
      settings: InternalSimscapePortConfiguration="{\"Bottom\":[],\"Left\":[{\"id\":\"A\",\"label\":\"\",\"type\":\"foundation.hydraulic.hydraulic\"}],\"Right\":[],\"Top\":[]}"
  Upper body R1 : fl_lib/Hydraulic/Hydraulic Elements/Linear Hydraulic Resistance  resistance=5.19e8 Pa/(m^3/s)  q_specify=off  q_priority=None  q=0.001 m^3/s  q_nominal_specify=off  q_nominal_unit=m^3/s  q_nominal_value=1  p_specify=off  p_priority=None  p=0 Pa  p_nominal_specify=off  p_nominal_unit=Pa  p_nominal_value=1
      settings: InternalSimscapePortConfiguration="{\"Bottom\":[],\"Left\":[{\"id\":\"A\",\"label\":\"A\",\"type\":\"foundation.hydraulic.hydraulic\"}],\"Right\":[{\"id\":\"B\",\"label\":\"B\",\"type\":\"foundation.hydraulic.hydraulic\"}],\"Top\":[]}"
  Upper body R2 : fl_lib/Hydraulic/Hydraulic Elements/Linear Hydraulic Resistance  resistance=0.31e8 Pa/(m^3/s)  q_specify=off  q_priority=None  q=0.001 m^3/s  q_nominal_specify=off  q_nominal_unit=m^3/s  q_nominal_value=1  p_specify=off  p_priority=None  p=0 Pa  p_nominal_specify=off  p_nominal_unit=Pa  p_nominal_value=1
      settings: InternalSimscapePortConfiguration="{\"Bottom\":[],\"Left\":[{\"id\":\"A\",\"label\":\"A\",\"type\":\"foundation.hydraulic.hydraulic\"}],\"Right\":[{\"id\":\"B\",\"label\":\"B\",\"type\":\"foundation.hydraulic.hydraulic\"}],\"Top\":[]}"
  Variable C Compliance Chamber{,1..2,5} (4 alike) : Cardiovascular_lib/Variable C Compliance Chamber  d_in=1e-2 m  length=1 m  time_const=0.01 s  k_sh=1.4  pressure_specify=off  pressure_priority=High  pressure=0 Pa  pressure_nominal_specify=off  pressure_nominal_unit=Pa  pressure_nominal_value=1  diameter_incr_specify=off  diameter_incr_priority=High  diameter_incr=0 m  diameter_incr_nominal_specify=off  diameter_incr_nominal_unit=m  diameter_incr_nominal_value=1  flow_rate_specify=off  flow_rate_priority=None  flow_rate=1e-3 m^3/s  flow_rate_nominal_specify=off  flow_rate_nominal_unit=m^3/s  flow_rate_nominal_value=1
      settings: InternalSimscapePortConfiguration="{\"Bottom\":[],\"Left\":[{\"id\":\"A\",\"label\":\"\",\"type\":\"foundation.hydraulic.hydraulic\"}],\"Right\":[{\"id\":\"V\",\"label\":\"C\",\"type\":\"input\"}],\"Top\":[]}"
  atrial check1 : sh_lib/Valves/Directional Valves/Check Valve  area_max=1e-1 m^2  pres_crack=0.01 Pa  pres_max=0.1 Pa  C_d=0.7  A_leak=1e-12 m^2  lam_spec=1  B_lam=0.999  Re_cr=12  dynamic=0  tau=0.1 s  area_init=1e-12 m^2
      settings: InternalSimscapePortConfiguration="{\"Bottom\":[],\"Left\":[{\"id\":\"A\",\"label\":\"A\",\"type\":\"foundation.hydraulic.hydraulic\"}],\"Right\":[{\"id\":\"B\",\"label\":\"B\",\"type\":\"foundation.hydraulic.hydraulic\"}],\"Top\":[]}"
  attempt : fl_lib/Physical Signals/Sources/PS Repeating Sequence  y_init=0  offset=0 s  sig_type=2  durations=[0.01 0.01 0.01 0.01 0.01 0.01 0.01 0.01 0.01 0.01 0.01 0.01 0.01 0.01 0.01 0.01 0.01 0.01 0.01 0.01 0.01 0.01 0.01 0.01 0.01 0.01 0.01 0.01 0.01 0.01 0.01 0.01 0.01 0.01 0.01 0.01 0.01 0.01 0.01 0.01 0.01 0.01 0.01 0.01 0.01 0.01 0.01 0.01 0.01 0.01 0.01 0.01 0.01 0.01 0.01 0.01 0.01 0.01 0.01 0.01 0.01 0.01 0.01 0.01 0.01 0.01 0.01 0.01 0.01 0.01 0.01 0.01 0.01 0.01 0.01 0.01 0.01 0.01 0.01 0.01 0.01 0.01 0.01 0.01 0.01 0.01 0.01 0.01 0.01 0.01 0.01 0.01 0.01 0.01 0.01 0.01 0.01 0.01 0.01 0.01] s  y_start="[1.00000000000000e-06\t9.37357264520457e-07\t8.74971941477825e-07\t8.13100385546094e-07\t7.51996840219996e-07\t6.91912393073946e-07\t6.33093943989338e-07\t5.75783190589981e-07\t5.20215635054710e-07\t4.66619616388422e-07\t4.15215372128128e-07\t3.66214133339669e-07\t3.19817256623959e-07\t2.76215396699523e-07\t2.35587722961358e-07\t1.98101183235464e-07\t1.63909817754413e-07\t1.33154126172990e-07\t1.05960490224980e-07\t8.24406543935084e-08\t6.26912667289963e-08\t4.67934817015874e-08\t3.48126267200239e-08\t2.67979336873100e-08\t2.27823366962635e-08\t2.27823366962635e-08\t2.67979336873100e-08\t3.48126267200239e-08\t4.67934817015874e-08\t6.26912667289962e-08\t8.24406543935083e-08\t1.05960490224980e-07\t1.33154126172990e-07\t1.63909817754413e-07\t1.98101183235464e-07\t2.35587722961358e-07\t2.76215396699523e-07\t3.19817256623959e-07\t3.66214133339669e-07\t4.15215372128128e-07\t4.66619616388422e-07\t5.20215635054710e-07\t5.75783190589981e-07\t6.33093943989338e-07\t6.91912393073945e-07\t7.51996840219996e-07\t8.13100385546094e-07\t8.74971941477825e-07\t9.37357264520457e-07\t1.00000000000000e-06\t1.00000000000000e-06\t1.00000000000000e-06\t1.00000000000000e-06\t1.00000000000000e-06\t1.00000000000000e-06\t1.00000000000000e-06\t1.00000000000000e-06\t1.00000000000000e-06\t1.00000000000000e-06\t1.00000000000000e-06\t1.00000000000000e-06\t1.00000000000000e-06\t1.00000000000000e-06\t1.00000000000000e-06\t1.00000000000000e-06\t1.00000000000000e-06\t1.00000000000000e-06\t1.00000000000000e-06\t1.00000000000000e-06\t1.00000000000000e-06\t1.00000000000000e-06\t1.00000000000000e-06\t1.00000000000000e-06\t1.00000000000000e-06\t1.00000000000000e-06\t1.00000000000000e-06\t1.00000000000000e-06\t1.00000000000000e-06\t1.00000000000000e-06\t1.00000000000000e-06\t1.50000000000000e-06\t1.50000000000000e-06\t1.50000000000000e-06\t1.50000000000000e-06\t1.50000000000000e-06\t1.50000000000000e-06\t1.50000000000000e-06\t1.50000000000000e-06\t1.50000000000000e-06\t1.50000000000000e-06\t1.50000000000000e-06\t1.50000000000000e-06\t1.50000000000000e-06\t1.50000000000000e-06\t1.50000000000000e-06\t1.50000000000000e-06\t1.50000000000000e-06\t1.50000000000000e-06\t1.50000000000000e-06\t1.50000000000000e-06]"  y_end=1
      settings: InternalSimscapePortConfiguration="{\"Bottom\":[],\"Left\":[],\"Right\":[{\"id\":\"Y\",\"label\":\"Y\",\"type\":\"output\"}],\"Top\":[]}"
  wires:
  PS-Simulink Converter1/1 -> Abdominal Scope4/1
  PS-Simulink Converter2/1 -> Abdominal Scope2/1
  PS-Simulink Converter4/1 -> Abdominal Scope3/1
  PS-Simulink Converter3/1 -> Abdominal Scope1/1
  PS-Simulink Converter5/1 -> Abdominal Scope5/1
  connections:
  LV pump/RConn1 -- Hydraulic Pressure Sensor1/LConn1 -- Hydraulic Pressure Sensor2/LConn1 -- "Blood "/RConn1 -- atrial check1/RConn1 -- LV/LConn1 -- Solver/RConn1
  Hydraulic Reference/LConn1 -- LV pump/RConn2
  Ideal Angular Velocity Source/LConn1 -- LV pump/LConn1
  Ideal Angular Velocity Source/RConn2 -- Mechanical Rotational Reference4/LConn1
  AV opening sequence/RConn1 -- Aortic valve/LConn1
  LV ejection sequence/RConn1 -- PS-Simulink Converter5/LConn1 -- Ideal Angular Velocity Source/RConn1
  LA filling sequence4/RConn1 -- Tricuspid valve/LConn1
  LV/RConn1 -- Hydraulic Pressure Sensor1/RConn1 -- Aortic valve/LConn2 -- Variable C Compliance Chamber5/LConn1
  Upper body R1/RConn1 -- Upper body C/LConn1 -- Upper body R2/LConn1
  Pulmonary R2/LConn1 -- Pulmonary C/LConn1 -- Pulmonary R1/RConn1
  PV opening sequence/RConn1 -- Pulmonary valve/LConn1
  LA filling sequence1/RConn1 -- Mitral/Bicuspid valve/LConn1
  Variable C Compliance Chamber1/RConn1 -- LA compliance2/RConn1
  Pulmonary R2/RConn1 -- Hydraulic Pressure Sensor3/LConn1 -- Aortic check 4/LConn1
  Abdominal R1/RConn1 -- Abdominal C/LConn1 -- Abdominal R2/LConn1
  Lower body R2/LConn1 -- Lower body C/LConn1 -- Lower body R1/RConn1
  Pulmonary artery/RConn1 -- Pulmonary R1/LConn1
  Lower body R1/LConn1 -- Hydraulic Pressure Sensor/LConn1 -- Abdominal R1/LConn1 -- Thoracic aorta/RConn1
  Descending aorta/LConn1 -- Upper body R1/LConn1 -- Ascending aorta/RConn1
  Thoracic aorta/LConn1 -- Descending aorta/RConn1
  RA check valve/LConn1 -- SVC/RConn1 -- Thoracic IVC/RConn1
  Upper body R2/RConn1 -- SVC/LConn1
  Abdominal R2/RConn1 -- Lower body R2/RConn1 -- Abdominal IVC/LConn1
  Abdominal IVC/RConn1 -- Hydraulic Pressure Sensor/RConn1 -- Thoracic IVC/LConn1
  Aortic check 4/RConn1 -- LA/LConn1
  Variable C Compliance Chamber2/RConn1 -- RV compliance sq/RConn1
  RV/RConn1 -- Variable C Compliance Chamber2/LConn1 -- Pulmonary valve/LConn2
  RA/RConn1 -- Variable C Compliance Chamber1/LConn1 -- Tricuspid valve/LConn2
  Aortic check 2/RConn1 -- Pulmonary artery/LConn1
  Mitral/Bicuspid valve/LConn2 -- Variable C Compliance Chamber/LConn1 -- LA/RConn1
  Tricuspid valve/RConn1 -- Aortic check 1/LConn1
  "Aortic check "/LConn1 -- Aortic valve/RConn1
  Ascending aorta/LConn1 -- Hydraulic Pressure Sensor2/RConn1 -- "Aortic check "/RConn1
  Pulmonary valve/RConn1 -- Hydraulic Pressure Sensor3/RConn1 -- Aortic check 2/LConn1
  RA/LConn1 -- RA check valve/RConn1
  Aortic check 1/RConn1 -- RV/LConn1
  Mitral/Bicuspid valve/RConn1 -- atrial check1/LConn1
  Variable C Compliance Chamber/RConn1 -- LA compliance1/RConn1
  Variable C Compliance Chamber5/RConn1 -- attempt/RConn1
  PS-Simulink Converter2/LConn1 -- Hydraulic Pressure Sensor1/RConn2
  PS-Simulink Converter1/LConn1 -- Hydraulic Pressure Sensor2/RConn2
  PS-Simulink Converter3/LConn1 -- Hydraulic Pressure Sensor/RConn2
  PS-Simulink Converter4/LConn1 -- Hydraulic Pressure Sensor3/RConn2
